simulink model "oddeven"  (R2021b)
settings: Solver=FixedStepDiscrete  StartTime=0.0  StopTime=10.0  RelTol=1e-3  EnableMultiTasking=on
settings Model: Creator=midol  LastModifiedBy=midol
settings DataIOCC: ReturnWorkspaceOutputs=off
settings OptimizationCC: DefaultParameterBehavior=Inlined  InlineInvariantSignals=on  EnableMemcpy=off  LifeSpan=1  EfficientTunableParamExpr=on
settings DebuggingCC: UnderspecifiedInitializationDetection=Classic  MergeDetectMultiDrivingBlocksExec=none  SFMachineParentedDataDiag=warning  ArithmeticOperatorsInVariantConditions=warning
settings ModelReferenceCC: PropagateSignalLabelsOutOfModel=off
settings SFSimCC: MATLABDynamicMemAlloc=off  CustomCodeUndefinedFunction=UseInterfaceOnly
settings RTWCC: Description=Embedded Coder  SystemTargetFile=ert.tlc  GenCodeOnly=on  TemplateMakefile=ert_default_tmf  GenerateReport=on  IncludeHyperlinkInReport=on  LaunchReport=on  GenerateTraceInfo=on  GenerateTraceReport=on  GenerateTraceReportSl=on  GenerateTraceReportSf=on  GenerateTraceReportEml=on
settings CodeAppCC: ForceParamTrailComments=on  IgnoreCustomStorageClasses=off  OperatorAnnotations=on  SimulinkDataObjDesc=on  SFDataObjDesc=on  MATLABFcnDesc=on  InsertBlockDesc=on  StateflowObjectComments=on  MATLABSourceComments=on
settings ERTTargetCC: MultiwordLength=2048  GenerateSampleERTMain=on  InlinedParameterPlacement=NonHierarchical  ERTCustomFileTemplate=example_file_process.tlc

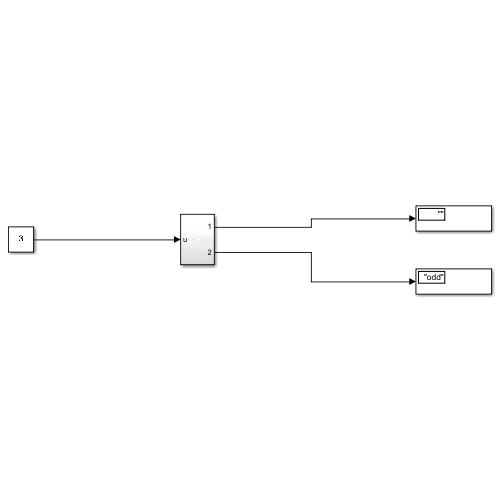
[thumbnail: Simulink's stored preview of the top-level diagram]
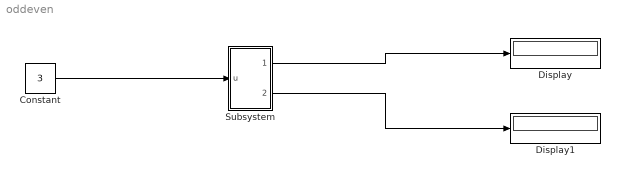
== system oddeven ==
  Constant : Constant  Value=3
  Display : Display
  Display1 : Display
  Subsystem : Subsystem
  wires:
  Constant/1 -> Subsystem/1(u)
  Subsystem/1(Out1) -> Display/1
  Subsystem/2(Out2) -> Display1/1

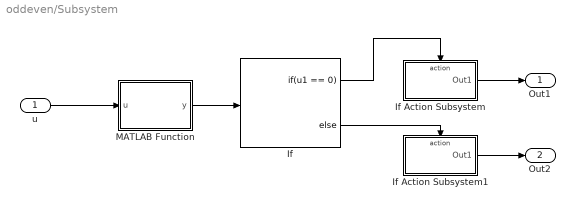
== system oddeven/Subsystem ==
  u : Inport
  If : If  IfExpression=u1 == 0
  If Action Subsystem : Subsystem  TreatAsAtomicUnit=on
  If Action Subsystem1 : Subsystem  TreatAsAtomicUnit=on
  MATLAB Function : MATLAB Function  TreatAsAtomicUnit=on
  Out1 : Outport
  Out2 : Outport  Port=2
  wires:
  u/1 -> MATLAB Function/1(u)
  MATLAB Function/1(y) -> If/1
  If/2 -> If Action Subsystem1/Action
  If Action Subsystem/1(Out1) -> Out1/1
  If/1 -> If Action Subsystem/Action
  If Action Subsystem1/1(Out1) -> Out2/1

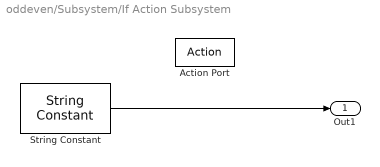
== system oddeven/Subsystem/If Action Subsystem ==
  Action Port : ActionPort  ActionPortLabel=if(u1 == 0)
  String Constant : StringConstant  String="\"even\""
  Out1 : Outport
  wires:
  String Constant/1 -> Out1/1

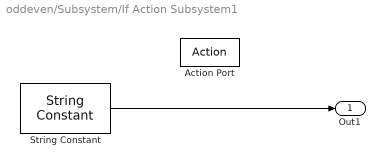
== system oddeven/Subsystem/If Action Subsystem1 ==
  Action Port : ActionPort  ActionPortLabel=else
  String Constant : StringConstant  String="\"odd\""
  Out1 : Outport
  wires:
  String Constant/1 -> Out1/1

== matlab function oddeven/Subsystem/MATLAB Function ==
  data: u input; y output
function y = fcn(u)

if(mod(u,2) == 0)
    y = 0;
else 
    y = 1;
end
